simulink model "flightControl"  (R2022a)
settings: Solver=VariableStepAuto  StartTime=0.0  StopTime=10.0  RelTol=1e-3
settings Model: Creator=willg  LastModifiedBy=willg

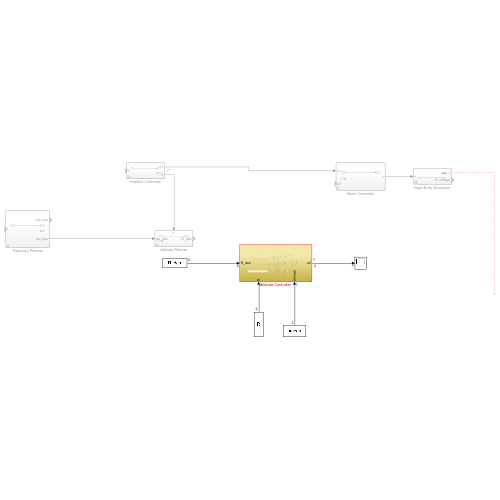
[thumbnail: Simulink's stored preview of the top-level diagram]
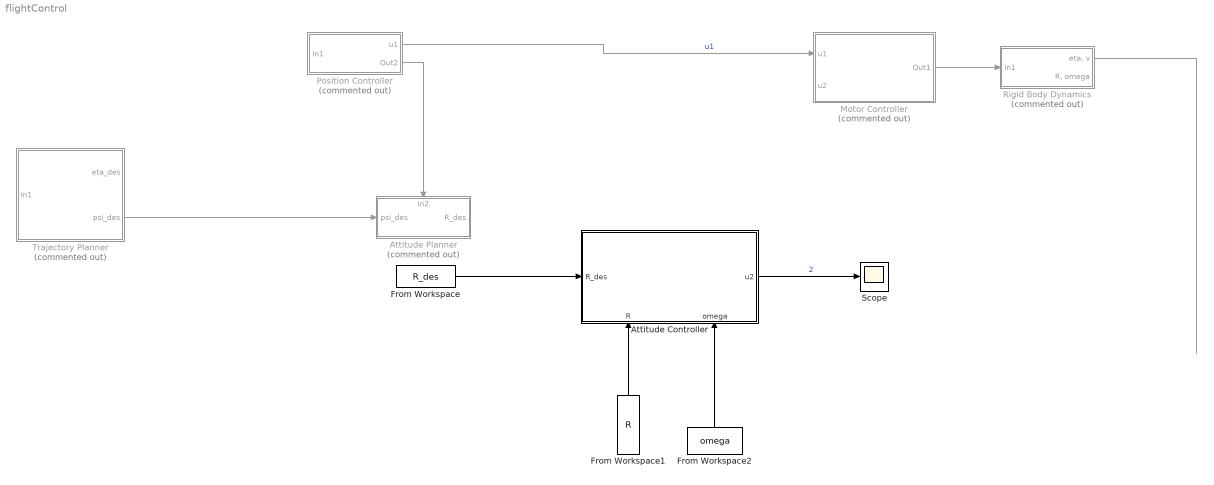
== system flightControl ==
  Attitude Controller : Subsystem
      settings: PortSchema="{\"entries\":[{\"content\":{\"sides\":[{\"content\":{\"connectorIds\":[\"In1\"]},\"type\":\"ConnectorPlacement.EquallySpacedRectSide\",\"uuid\":\"630ecae2-e1db-4b8a-a9a2-183b48bc47da\"},{\"content\":{\"connectorIds\":[\"Out1\"],\"side\":\"RIGHT\"},\"type\":\"ConnectorPlacement.EquallySpacedRectSide\",\"uuid\":\"e904aa9f-458e-4bff-a993-74555f26f12b\"},{\"content\":{\"connectorIds\":[],\"side\":\"TOP\"},\"type\":\"ConnectorPlacement.EquallySpacedRectSide\",\"uuid\":\"30bd5434-3545-4347-b0b8-6517da3f1f1d\"},{\"content\":{\"connectorIds\":[\"In2\",\"In3\"],\"side\":\"BOTTOM\"},\"type\":\"ConnectorPlacement.EquallySpacedRectSide\",\"uuid\":\"b84fc4fd-1ce7-4a26-859c-fab4b37ef513\"}]},\"type\":\"ConnectorPlacement.EquallySpacedConnector\",\"uuid\":\"25596745-a1e3-46c8-a956-00323e342a37\"}],\"packageUris\":[\"http://schema.mathworks.com/mf0/Connector/R2020b\"],\"version\":\"1.0\"}"
  Attitude Planner : Subsystem  Commented=on
      settings: PortSchema="{\"entries\":[{\"content\":{\"sides\":[{\"content\":{\"connectorIds\":[\"In1\"]},\"type\":\"ConnectorPlacement.EquallySpacedRectSide\",\"uuid\":\"630ecae2-e1db-4b8a-a9a2-183b48bc47da\"},{\"content\":{\"connectorIds\":[\"Out1\"],\"side\":\"RIGHT\"},\"type\":\"ConnectorPlacement.EquallySpacedRectSide\",\"uuid\":\"e904aa9f-458e-4bff-a993-74555f26f12b\"},{\"content\":{\"connectorIds\":[\"In2\"],\"side\":\"TOP\"},\"type\":\"ConnectorPlacement.EquallySpacedRectSide\",\"uuid\":\"30bd5434-3545-4347-b0b8-6517da3f1f1d\"}]},\"type\":\"ConnectorPlacement.EquallySpacedConnector\",\"uuid\":\"25596745-a1e3-46c8-a956-00323e342a37\"}],\"packageUris\":[\"http://schema.mathworks.com/mf0/Connector/R2020b\"],\"version\":\"1.0\"}"
  From Workspace : FromWorkspace  VariableName=R_des
  From Workspace1 : FromWorkspace  VariableName=R
  From Workspace2 : FromWorkspace  VariableName=omega
  Motor Controller : Subsystem  Commented=on
  Position Controller : Subsystem  Commented=on
  Rigid Body Dynamics : Subsystem  Commented=on
  Scope : Scope
  Trajectory Planner : Subsystem  Commented=on
  wires:
  Motor Controller/1(Out1) -> Rigid Body Dynamics/1(In1)
  Position Controller/1(u1) -> Motor Controller/1(u1)  "u1"
  Rigid Body Dynamics/1("eta, v") -> ?
  Position Controller/2(Out2) -> Attitude Planner/2(In2)
  Trajectory Planner/2(psi_des) -> Attitude Planner/1(psi_des)
  From Workspace/1 -> Attitude Controller/1(R_des)
  Attitude Controller/1(u2) -> Scope/1  "2"
  From Workspace1/1 -> Attitude Controller/2(R)
  From Workspace2/1 -> Attitude Controller/3(omega)

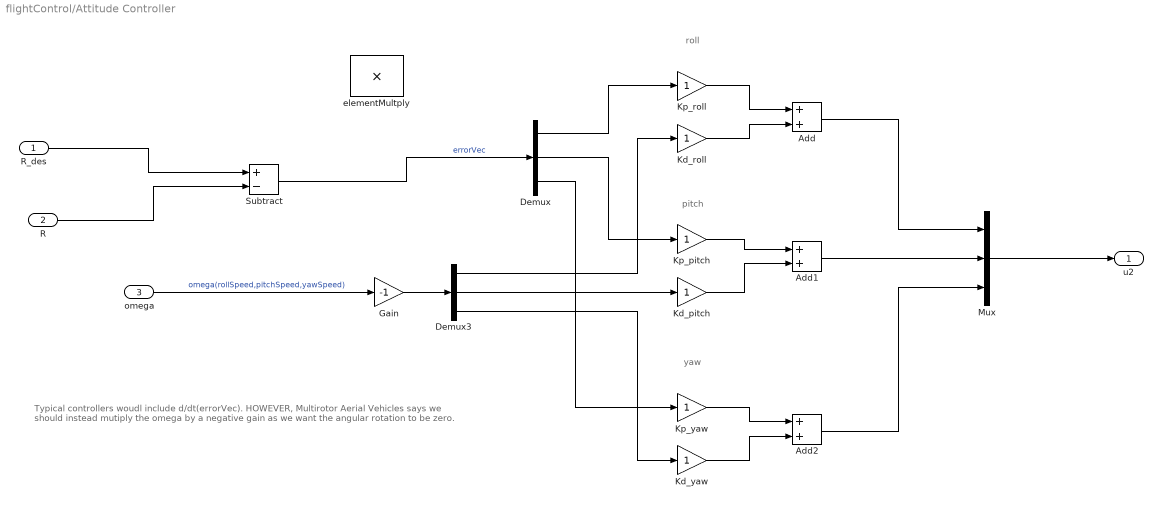
== system flightControl/Attitude Controller ==
  note: Typical controllers woudl include d/dt(errorVec). HOWEVER, Multirotor Aerial Vehicles says we should instead mutiply the omega by a negative gain as we want the angular rotation to be zero.
  note: roll
  note: pitch
  note: yaw
  R_des : Inport
  R : Inport  Port=2
  omega : Inport  Port=3
  Add : Sum
  Add1 : Sum
  Add2 : Sum
  Demux : Demux  Outputs=3
  Demux3 : Demux  Outputs=3
  Gain : Gain  Gain=-1
  Kd_pitch : Gain
  Kd_roll : Gain
  Kd_yaw : Gain
  Kp_pitch : Gain
  Kp_roll : Gain
  Kp_yaw : Gain
  Mux : Mux  Inputs=3
  Subtract : Sum  Inputs=+-
  "elementMultply " : Product
  u2 : Outport
  wires:
  R_des/1 -> Subtract/1
  Kp_roll/1 -> Add/1
  Kd_roll/1 -> Add/2
  Subtract/1 -> Demux/1  "errorVec"
  omega/1 -> Gain/1  "omega(rollSpeed,pitchSpeed,yawSpeed)"
  Gain/1 -> Demux3/1
  Demux/1 -> Kp_roll/1
  Demux/2 -> Kp_pitch/1
  Demux/3 -> Kp_yaw/1
  Demux3/1 -> Kd_roll/1
  Demux3/2 -> Kd_pitch/1
  Demux3/3 -> Kd_yaw/1
  Kp_yaw/1 -> Add2/1
  Kd_yaw/1 -> Add2/2
  Kp_pitch/1 -> Add1/1
  Kd_pitch/1 -> Add1/2
  Add1/1 -> Mux/2
  Add/1 -> Mux/1
  Add2/1 -> Mux/3
  Mux/1 -> u2/1
  R/1 -> Subtract/2

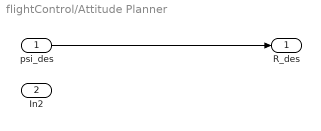
== system flightControl/Attitude Planner ==
  psi_des : Inport
  In2 : Inport  Port=2
  R_des : Outport
  wires:
  psi_des/1 -> R_des/1

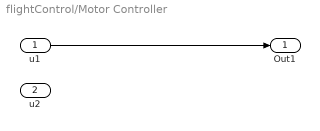
== system flightControl/Motor Controller ==
  u1 : Inport
  u2 : Inport  Port=2
  Out1 : Outport
  wires:
  u1/1 -> Out1/1

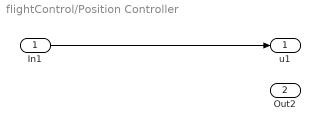
== system flightControl/Position Controller ==
  In1 : Inport
  u1 : Outport
  Out2 : Outport  Port=2
  wires:
  In1/1 -> u1/1

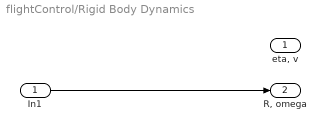
== system flightControl/Rigid Body Dynamics ==
  In1 : Inport
  "eta, v" : Outport
  "R, omega" : Outport  Port=2
  wires:
  In1/1 -> "R, omega"/1

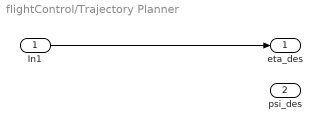
== system flightControl/Trajectory Planner ==
  In1 : Inport
  eta_des : Outport
  psi_des : Outport  Port=2
  wires:
  In1/1 -> eta_des/1
